simulink model "DCMLab2"  (R2021a)
settings: Solver=VariableStepAuto  StartTime=0.0  StopTime=5  RelTol=1e-3
libraries: spsSeriesRLCBranchLib x10, spsMeanLib x10, spsCurrentMeasurementLib x6, spsDCVoltageSourceLib x4, spsIdealSwitchLib x4, spsVoltageMeasurementLib x4, spsDiodeLib x3, spspowerguiLib x1
settings Model: Creator=manram  LastModifiedBy=manram

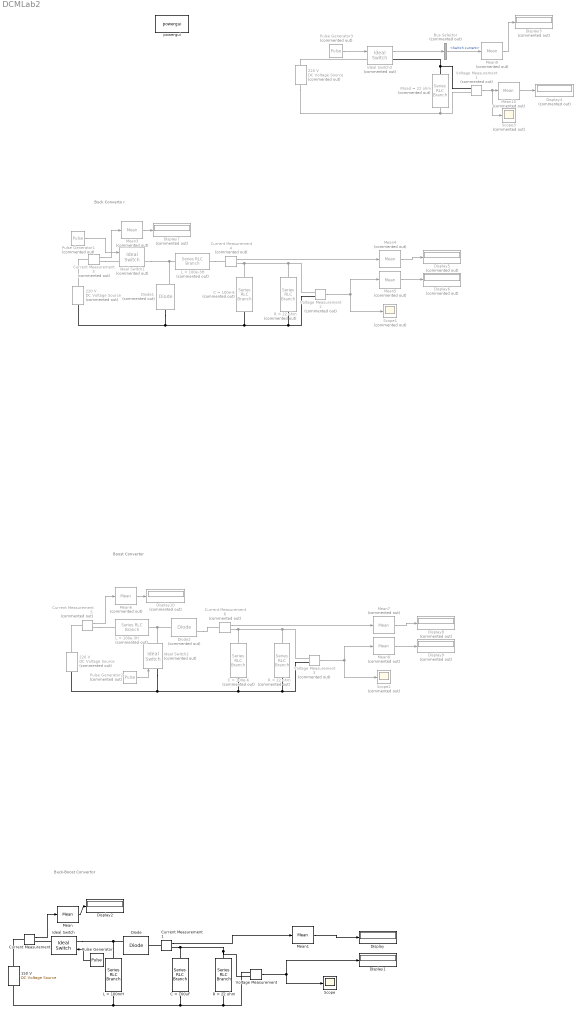
== system DCMLab2 ==
  note: Buck-Boost Convertor
  note: Boost Convertor
  note: Buck Converto r
  150 V : spsDCVoltageSourceLib/DC Voltage Source  Amplitude=150  Measurements=None
  220 V : spsDCVoltageSourceLib/DC Voltage Source  Commented=on  Amplitude=220  Measurements=None
  "220 V  " : spsDCVoltageSourceLib/DC Voltage Source  Commented=on  Amplitude=220  Measurements=None
  "220 V    " : spsDCVoltageSourceLib/DC Voltage Source  Commented=on  Amplitude=220  Measurements=None
  Bus Selector : BusSelector  Commented=on  OutputSignals=Switch current
  C = 100e-6 : spsSeriesRLCBranchLib/Series RLC Branch  Commented=on  LConnTagsString=__new0  RConnTagsString=__new0  BranchType=C  Resistance=1  Inductance=1e-3  SetiL0=off  InitialCurrent=0  Capacitance=100e-6  Setx0=off  InitialVoltage=0  Measurements=None
  "C = 100e-6     " : spsSeriesRLCBranchLib/Series RLC Branch  Commented=on  LConnTagsString=__new0  RConnTagsString=__new0  BranchType=C  Resistance=1  Inductance=1e-3  SetiL0=off  InitialCurrent=0  Capacitance=100e-6  Setx0=off  InitialVoltage=0  Measurements=None
  C = 100uF : spsSeriesRLCBranchLib/Series RLC Branch  LConnTagsString=__new0  RConnTagsString=__new0  BranchType=C  Resistance=1  Inductance=1e-3  SetiL0=off  InitialCurrent=0  Capacitance=100e-6  Setx0=off  InitialVoltage=0  Measurements=None
  Current Measurement : spsCurrentMeasurementLib/Current Measurement  PhasorSimulation=off  OutputType=Complex  PSBequivalent=0
  Current Measurement1 : spsCurrentMeasurementLib/Current Measurement  PhasorSimulation=off  OutputType=Complex  PSBequivalent=0
  Current Measurement{3..6} (4 alike) : spsCurrentMeasurementLib/Current Measurement  Commented=on  PhasorSimulation=off  OutputType=Complex  PSBequivalent=0
  Diode : spsDiodeLib/Diode  Ron=0.001  Lon=0  Vf=0.8  IC=0  UseSnubber=0  Rs=500  Cs=250e-9  Measurements=on
  Diode1 : spsDiodeLib/Diode  Commented=on  Ron=0.001  Lon=0  Vf=0.8  IC=0  UseSnubber=0  Rs=500  Cs=250e-9  Measurements=on
  Diode2 : spsDiodeLib/Diode  Commented=on  Ron=0.001  Lon=0  Vf=0.8  IC=0  UseSnubber=0  Rs=500  Cs=250e-9  Measurements=on
  Display : Display
  Display1 : Display
  Display{3..10} (8 alike) : Display  Commented=on
  Display2 : Display
  Ideal Switch : spsIdealSwitchLib/Ideal Switch  Ron=0.001  Lon=0  IC=0  Rs=1e5  Cs=inf  Measurements=on
  Ideal Switch1 : spsIdealSwitchLib/Ideal Switch  Commented=on  Ron=0.001  Lon=0  IC=0  Rs=1e5  Cs=inf  Measurements=on
  Ideal Switch2 : spsIdealSwitchLib/Ideal Switch  Commented=on  Ron=0.001  Lon=0  IC=0  Rs=1e5  Cs=inf  Measurements=on
  Ideal Switch3 : spsIdealSwitchLib/Ideal Switch  Commented=on  Ron=0.001  Lon=0  IC=0  Rs=1e5  Cs=inf  Measurements=on
  L = 100e-3H : spsSeriesRLCBranchLib/Series RLC Branch  Commented=on  LConnTagsString=__new0  RConnTagsString=__new0  BranchType=L  Resistance=1  Inductance=100e-3  SetiL0=off  InitialCurrent=0  Capacitance=1e-6  Setx0=off  InitialVoltage=0  Measurements=None
  "L = 100e-3H   " : spsSeriesRLCBranchLib/Series RLC Branch  Commented=on  LConnTagsString=__new0  RConnTagsString=__new0  BranchType=L  Resistance=1  Inductance=100e-3  SetiL0=off  InitialCurrent=0  Capacitance=1e-6  Setx0=off  InitialVoltage=0  Measurements=None
  L = 100mH : spsSeriesRLCBranchLib/Series RLC Branch  LConnTagsString=__new0  RConnTagsString=__new0  BranchType=L  Resistance=1  Inductance=0.1  SetiL0=off  InitialCurrent=0  Capacitance=1e-6  Setx0=off  InitialVoltage=0  Measurements=None
  Mean : spsMeanLib/Mean  Freq=1  Vinit=0  Ts=0
  Mean1 : spsMeanLib/Mean  Freq=10e3  Vinit=0  Ts=0
  Mean{6..10} (5 alike) : spsMeanLib/Mean  Commented=on  Freq=1  Vinit=0  Ts=0
  Mean3 : spsMeanLib/Mean  Commented=on  Freq=60  Vinit=0  Ts=0
  Mean4 : spsMeanLib/Mean  Commented=on  Freq=60  Vinit=0  Ts=0
  Mean5 : spsMeanLib/Mean  Commented=on  Freq=60  Vinit=0  Ts=0
  Pulse Generator : DiscretePulseGenerator  PulseType=Time based  Period=1/10000  PulseWidth=50
  Pulse Generator1 : DiscretePulseGenerator  Commented=on  PulseType=Time based  Period=1/10000  PulseWidth=50
  Pulse Generator2 : DiscretePulseGenerator  Commented=on  PulseType=Time based  Period=1/10000  PulseWidth=50
  Pulse Generator3 : DiscretePulseGenerator  Commented=on  PulseType=Time based  Period=1  PulseWidth=50
  R = 22 ohm : spsSeriesRLCBranchLib/Series RLC Branch  LConnTagsString=__new0  RConnTagsString=__new0  BranchType=R  Resistance=22  Inductance=1e-3  SetiL0=off  InitialCurrent=0  Capacitance=1e-6  Setx0=off  InitialVoltage=0  Measurements=None
  "R = 22 ohm   " : spsSeriesRLCBranchLib/Series RLC Branch  Commented=on  LConnTagsString=__new0  RConnTagsString=__new0  BranchType=R  Resistance=22  Inductance=1e-3  SetiL0=off  InitialCurrent=0  Capacitance=1e-6  Setx0=off  InitialVoltage=0  Measurements=None
  "R = 22 ohm    " : spsSeriesRLCBranchLib/Series RLC Branch  Commented=on  LConnTagsString=__new0  RConnTagsString=__new0  BranchType=R  Resistance=22  Inductance=1e-3  SetiL0=off  InitialCurrent=0  Capacitance=1e-6  Setx0=off  InitialVoltage=0  Measurements=None
  "Rload = 22 ohm " : spsSeriesRLCBranchLib/Series RLC Branch  Commented=on  LConnTagsString=__new0  RConnTagsString=__new0  BranchType=R  Resistance=22  Inductance=1e-3  SetiL0=off  InitialCurrent=0  Capacitance=1e-6  Setx0=off  InitialVoltage=0  Measurements=None
  Scope : Scope
  Scope1 : Scope  Commented=on
  Scope2 : Scope  Commented=on
  Scope3 : Scope  Commented=on
  Voltage Measurement : spsVoltageMeasurementLib/Voltage Measurement  PhasorSimulation=off  OutputType=Complex  PSBequivalent=0
  Voltage Measurement1 : spsVoltageMeasurementLib/Voltage Measurement  Commented=on  PhasorSimulation=off  OutputType=Complex  PSBequivalent=0
  Voltage Measurement2 : spsVoltageMeasurementLib/Voltage Measurement  Commented=on  PhasorSimulation=off  OutputType=Complex  PSBequivalent=0
  Voltage Measurement3 : spsVoltageMeasurementLib/Voltage Measurement  Commented=on  PhasorSimulation=off  OutputType=Complex  PSBequivalent=0
  powergui : spspowerguiLib/powergui  Priority=1  SimulationMode=Continuous  SampleTime=50e-6  frequency=60  Iterations=50  frequencyindice=0  Pbase=100e6  ErrMax=1e-4  UnitsV=kV  UnitsW=MW  buscounter=0  FunctionMessages=off  echomessages=off  EnableUseOfTLC=off  CurrentSourceSwitches=off  DisableSnubberDevices=off  DisableRonSwitches=off  DisableVfSwitches=off  DisplayEquations=off  AutomaticDiscreteSolvers=off  SolverType=Tustin/Backward Euler (TBE)  Interpol=off  ExternalGateDelay=off  methode=off  Ts=100  x0status=zero  SPID=on  SwTol=0  HookPort=off  NonlinearTolerance=1e-4  nMaxIteration=100  ContinueOnMaxIteration=off  RestoreLinks=warning  ResistiveCurrentMeasurement=off  Frange=[0:2:500]  Ylog=off  Xlog=on  ShowGrid=off  save=off  variable=ZData  structure=0  ZoomFFT=off  StartTime=0.0  cycles=1  DisplayStyle=1  fundamental=60  FreqAxis=off  MaxFrequency=1000  frequencyindicesteady=1  RmsSteady=1  display=off
  wires:
  Pulse Generator/1 -> Ideal Switch/1
  Mean/1 -> Display2/1
  Current Measurement/1 -> Mean/1
  Voltage Measurement1/1 -> Scope3/1, Mean10/1
  Mean9/1 -> Display3/1
  Voltage Measurement2/1 -> Scope1/1, Mean5/1
  Mean5/1 -> Display6/1
  Mean3/1 -> Display7/1
  Current Measurement4/1 -> Mean4/1
  Mean4/1 -> Display5/1
  Current Measurement3/1 -> Mean3/1
  Pulse Generator1/1 -> Ideal Switch1/1
  Pulse Generator2/1 -> Ideal Switch2/1
  Voltage Measurement3/1 -> Scope2/1, Mean8/1
  Mean8/1 -> Display9/1
  Mean6/1 -> Display10/1
  Current Measurement5/1 -> Mean6/1
  Mean7/1 -> Display8/1
  Current Measurement6/1 -> Mean7/1
  Ideal Switch3/1 -> Bus Selector/1
  Bus Selector/1 -> Mean9/1  "<Switch current>"
  Pulse Generator3/1 -> Ideal Switch3/1
  Mean10/1 -> Display4/1
  Mean1/1 -> Display/1
  Voltage Measurement/1 -> Display1/1, Scope/1
  Current Measurement1/1 -> Mean1/1
  connections:
  L = 100mH/RConn1 -- 150 V/LConn1 -- C = 100uF/LConn1 -- Voltage Measurement/LConn1 -- R = 22 ohm/RConn1
  Diode/RConn1 -- Ideal Switch/LConn1 -- L = 100mH/LConn1
  Current Measurement1/RConn1 -- Voltage Measurement/LConn2 -- R = 22 ohm/LConn1 -- C = 100uF/RConn1
  Current Measurement/LConn1 -- 150 V/RConn1
  Current Measurement1/LConn1 -- Diode/LConn1
  220 V/RConn1 -- Ideal Switch3/LConn1
  "Rload = 22 ohm "/LConn1 -- Ideal Switch3/RConn1 -- Voltage Measurement1/LConn1
  220 V/LConn1 -- Voltage Measurement1/LConn2 -- "Rload = 22 ohm "/RConn1
  Voltage Measurement2/LConn1 -- "R = 22 ohm   "/LConn1 -- C = 100e-6/LConn1 -- Current Measurement4/RConn1
  C = 100e-6/RConn1 -- Diode1/LConn1 -- "220 V  "/LConn1 -- Voltage Measurement2/LConn2 -- "R = 22 ohm   "/RConn1
  Current Measurement3/LConn1 -- "220 V  "/RConn1
  L = 100e-3H/LConn1 -- Current Measurement4/LConn1
  Current Measurement3/RConn1 -- Ideal Switch1/LConn1
  L = 100e-3H/RConn1 -- Diode1/RConn1 -- Ideal Switch1/RConn1
  Voltage Measurement3/LConn1 -- "R = 22 ohm    "/LConn1 -- "C = 100e-6     "/LConn1 -- Current Measurement6/RConn1
  "C = 100e-6     "/RConn1 -- Voltage Measurement3/LConn2 -- "R = 22 ohm    "/RConn1 -- "220 V    "/LConn1 -- Ideal Switch2/LConn1
  Current Measurement5/LConn1 -- "220 V    "/RConn1
  Current Measurement5/RConn1 -- "L = 100e-3H   "/RConn1
  Diode2/LConn1 -- Ideal Switch2/RConn1 -- "L = 100e-3H   "/LConn1
  Diode2/RConn1 -- Current Measurement6/LConn1
  Ideal Switch/RConn1 -- Current Measurement/RConn1
